simulink model "transmitancje_model"  (R2015a)
settings: Solver=ode45  StartTime=0.0  StopTime=czas_sym  MaxStep=tmax  RelTol=1e-3
values from neighbouring files (symbols this model uses):
  dQg = QgN*0.1    [dokladny.m]    (also in kupfmuller.m; row_stanu.m; ss_tf.m; transmitancje.m = QgN*0.0)
  dTzew = 0    [dokladny.m]    (also in kupfmuller.m; row_stanu.m; ss_tf.m = 2; transmitancje.m = 2)
  L11 = [ Cvs*MTw,              - Kw^2 + MTw*Kw + Ks*MTw]    [ss_tf_support.m]    (also in transmitancje.m; z_rownania.m = fliplr(coeffs(L1Qg, s)))
  L12 = [ Cvs*Kg*P,              Kg*Ks*Kw + Kg*Ks*P + Kg*Kw*P]    [ss_tf_support.m]    (also in transmitancje.m; z_rownania.m = fliplr(coeffs(L1Tz, s)))
  L21 = [ Kg*Kw]    [ss_tf_support.m]    (also in transmitancje.m; z_rownania.m = fliplr(coeffs(L2Qg, s)))
  L22 = [ Cvg*Ks*MTw + Cvg*Kw*P,              Kg*Ks*MTw - Kg^2*Ks + Kg*Kw*P]    [ss_tf_support.m]    (also in transmitancje.m; z_rownania.m = fliplr(coeffs(L2Tz, s)))
  L31 = [ Cvs*Kg,              Kg*Ks + Kg*Kw]    [ss_tf_support.m]    (also in transmitancje.m; z_rownania.m = fliplr(coeffs(L3Qg, s)))
  L32 = [ Cvg*Cvs*P,  Cvg*Ks*Kw + Cvs*Kg*P + Cvg*Ks*P + Cvg*Kw*P,               Kg*Ks*Kw + Kg*Ks*P + Kg*Kw*P]    [ss_tf_support.m]    (also in transmitancje.m; z_rownania.m = fliplr(coeffs(L3Tz, s)))
  M = [ Cvg*Cvs*MTw,           - Cvs*Kg^2 + Cvs*MTw*Kg - Cvg*Kw^2 + Cvg*MTw*Kw + Cvg*Ks*MTw,           Kg*(-Kg*Kw - Ks*Kg - Kw^2 + MTw*Kw + Ks*MTw)]    [ss_tf_support.m]    (also in transmitancje.m; z_rownania.m = fliplr(coeffs(M1, s)))
  t0 = 40000    [dokladny.m]    (also in kupfmuller.m; row_stanu.m; transmitancje.m)
  Tg0 = -(Ks*MTw*Qg0 - Kw^2*Qg0 + Kw*MTw*Qg0 + P*Kg*Ks*Tzew0 + P*Kg*Kw*Tzew0 + Kg*Ks*Kw*Tzew0)/(Kg*(Kw^2 + Kg*Ks + Kg*Kw - Ks*MTw - Kw*MTw))    [dokladny.m]    (also in kupfmuller.m; row_stanu.m; ss_tf_support.m; transmitancje.m)
  Ts0 = -(Kw*Qg0 + P*Kw*Tzew0 - Kg*Ks*Tzew0 + Ks*MTw*Tzew0)/(Kw^2 + Kg*Ks + Kg*Kw - Ks*MTw - Kw*MTw)    [dokladny.m]    (also in kupfmuller.m; row_stanu.m; ss_tf_support.m; transmitancje.m)
  Twew0 = -(Ks*Qg0 + Kw*Qg0 + Ks*Kw*Tzew0 + Ks*P*Tzew0 + Kw*P*Tzew0)/(Kw^2 + Kg*Ks + Kg*Kw - Ks*MTw - Kw*MTw)    [dokladny.m]    (also in kupfmuller.m; row_stanu.m; transmitancje.m)
settings Model: Creator=Prezes  LastModifiedBy=Prezes

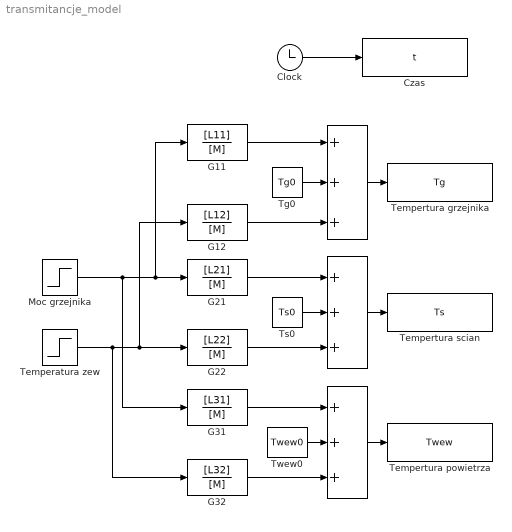
== system transmitancje_model ==
  " " : Sum  Inputs=+++
  "   " : Sum  Inputs=+++
  " " : Sum  Inputs=+++
  Clock : Clock
  Czas : ToWorkspace  VariableName=t  SampleTime=-1
      settings: Save2DSignal=2-D array (concatenate along first dimension)
  G11 : TransferFcn  Numerator=[L11]  Denominator=[M]
  G12 : TransferFcn  Numerator=[L12]  Denominator=[M]
  G21 : TransferFcn  Numerator=[L21]  Denominator=[M]
  G22 : TransferFcn  Numerator=[L22]  Denominator=[M]
  G31 : TransferFcn  Numerator=[L31]  Denominator=[M]
  G32 : TransferFcn  Numerator=[L32]  Denominator=[M]
  Moc grzejnika : Step  Time=t0  After=dQg  SampleTime=0
  Temperatura zew : Step  Time=t0  After=dTzew  SampleTime=0
  Tempertura grzejnika : ToWorkspace  VariableName=Tg  SampleTime=-1
      settings: Save2DSignal=2-D array (concatenate along first dimension)
  Tempertura powietrza : ToWorkspace  VariableName=Twew  SampleTime=-1
      settings: Save2DSignal=2-D array (concatenate along first dimension)
  Tempertura scian : ToWorkspace  VariableName=Ts  SampleTime=-1
      settings: Save2DSignal=2-D array (concatenate along first dimension)
  Tg0 : Constant  Value=Tg0
  Ts0 : Constant  Value=Ts0
  Twew0 : Constant  Value=Twew0
  wires:
  Clock/1 -> Czas/1
  G11/1 -> " "/1
  G21/1 -> "   "/1
  Moc grzejnika/1 -> G11/1, G21/1, G31/1
  Temperatura zew/1 -> G12/1, G22/1, G32/1
  "   "/1 -> Tempertura scian/1
  " "/1 -> Tempertura grzejnika/1
  Ts0/1 -> "   "/2
  G22/1 -> "   "/3
  G12/1 -> " "/3
  Tg0/1 -> " "/2
  G31/1 -> " "/1
  " "/1 -> Tempertura powietrza/1
  Twew0/1 -> " "/2
  G32/1 -> " "/3
